simulink model "simulink_sfunt_fuzzy_"  (R2022b)
settings: Solver=VariableStepAuto  StartTime=0.0  StopTime=30  RelTol=1e-3
libraries: fuzblock x1
settings Model: Creator=23776  LastModifiedBy=23776

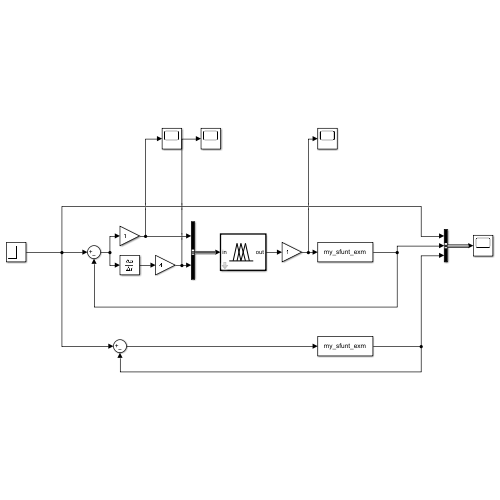
[thumbnail: Simulink's stored preview of the top-level diagram]
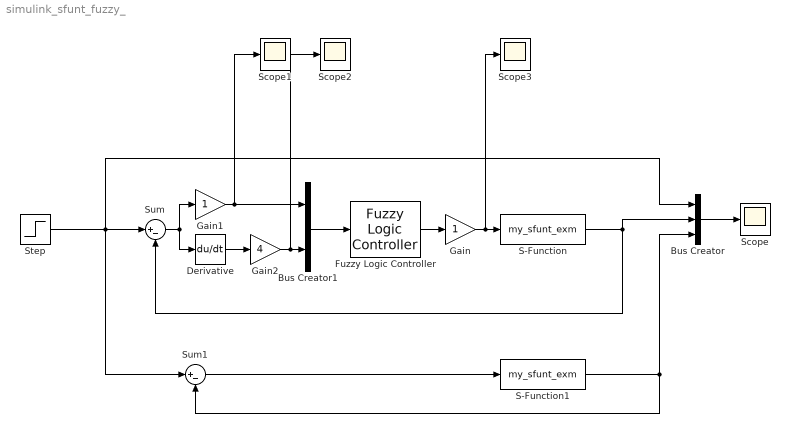
== system simulink_sfunt_fuzzy_ ==
  Bus Creator : BusCreator  Inputs=3
  Bus Creator1 : BusCreator  Inputs=2
  Derivative : Derivative
  Fuzzy Logic Controller : fuzblock/Fuzzy Logic  Controller  FIS='Fuzzy_Test.fis'  OutputSampleNumber=101  DataType=double  FuzzifiedInputs=off  RuleFiringStrengths=off  RuleOutputs=off  AggregatedOutputs=off  SimulateUsing=Interpreted execution  OutOfRangeInputValueMessage=warning  NoRuleFiredMessage=warning  EmptyOutputFuzzySetMessage=warning
  Gain : Gain
  Gain1 : Gain
  Gain2 : Gain  Gain=4
  S-Function : S-Function  FunctionName=my_sfunt_exm  SFunctionDeploymentMode=off  EnableBusSupport=off
  S-Function1 : S-Function  FunctionName=my_sfunt_exm  SFunctionDeploymentMode=off  EnableBusSupport=off
  Scope{,1..3} (4 alike) : Scope
  Step : Step  SampleTime=0
  Sum : Sum  Inputs=|+-
  Sum1 : Sum  Inputs=|+-
  wires:
  Bus Creator/1 -> Scope/1
  Step/1 -> Sum1/1, Sum/1, Bus Creator/1
  S-Function/1 -> Sum/2, Bus Creator/2
  Bus Creator1/1 -> Fuzzy Logic Controller/1
  Fuzzy Logic Controller/1 -> Gain/1
  Gain/1 -> Scope3/1, S-Function/1
  Gain1/1 -> Bus Creator1/1, Scope1/1
  Gain2/1 -> Scope2/1, Bus Creator1/2
  Sum/1 -> Derivative/1, Gain1/1
  Sum1/1 -> S-Function1/1
  S-Function1/1 -> Bus Creator/3, Sum1/2
  Derivative/1 -> Gain2/1
